simulink model "lyskawaLab6_si_nonlinear"  (R2023b)
settings: Solver=VariableStepAuto  StartTime=0.0  StopTime=stopTime  MaxStep=0.01  RelTol=1e-3
values from neighbouring files (symbols this model uses):
  A1 = 2    [lyskawaLab6.m]
  A2 = 6    [lyskawaLab6.m]
  Aw1 = 0.1 * 2    (= 0.2)    [lyskawaLab6.m]
  Aw2 = 0.1 * 6    (= 0.6)    [lyskawaLab6.m]
  dfwe1 = 0.1*fwe1max    [lyskawaLab6.m]
  dfwe2 = 0    [lyskawaLab6.m]
  fwe1_0 = arrayfwe1_0(i)    [lyskawaLab6.m]
  fwe2_0 = 0.1 * fwe2max    [lyskawaLab6.m]
  g = 9.81    [lyskawaLab6.m]
  h1_0 = fwe1_0^2/(Aw1^2 *2*g)    [lyskawaLab6.m]
  h2_0 = (fwe1_0 + fwe2_0)^2/(Aw2^2 * 2*g)    [lyskawaLab6.m]
  t0 = 5    [lyskawaLab6.m]
settings Model: Creator=aleklyskawa  LastModifiedBy=aleklyskawa

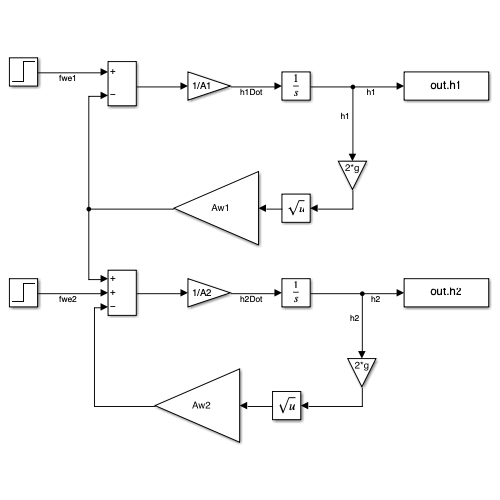
[thumbnail: Simulink's stored preview of the top-level diagram]
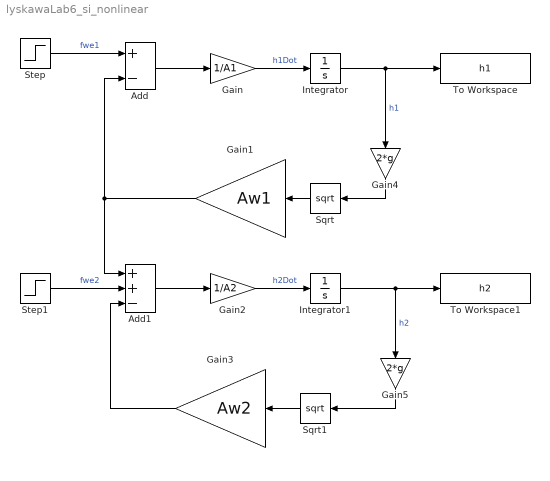
== system lyskawaLab6_si_nonlinear ==
  Add : Sum  Inputs=+-
  Add1 : Sum  Inputs=++-
  Gain : Gain  Gain=1/A1
  Gain1 : Gain  Gain=Aw1
  Gain2 : Gain  Gain=1/A2
  Gain3 : Gain  Gain=Aw2
  Gain4 : Gain  Gain=2*g
  Gain5 : Gain  Gain=2*g
  Integrator : Integrator  InitialCondition=h1_0
  Integrator1 : Integrator  InitialCondition=h2_0
  Sqrt : Sqrt
  Sqrt1 : Sqrt
  Step : Step  Time=t0  Before=fwe1_0  After=fwe1_0 + dfwe1  SampleTime=0
  Step1 : Step  Time=t0  Before=fwe2_0  After=fwe2_0 + dfwe2  SampleTime=0
  To Workspace : ToWorkspace  VariableName=h1  SampleTime=-1
  To Workspace1 : ToWorkspace  VariableName=h2  SampleTime=-1
  wires:
  Gain1/1 -> Add/2, Add1/1
  Gain2/1 -> Integrator1/1  "h2Dot"
  Add1/1 -> Gain2/1
  Integrator/1 -> Gain4/1, To Workspace/1  "h1"
  Integrator1/1 -> Gain5/1, To Workspace1/1  "h2"
  Step1/1 -> Add1/2  "fwe2"
  Gain/1 -> Integrator/1  "h1Dot"
  Add/1 -> Gain/1
  Step/1 -> Add/1  "fwe1"
  Sqrt/1 -> Gain1/1
  Sqrt1/1 -> Gain3/1
  Gain3/1 -> Add1/3
  Gain4/1 -> Sqrt/1
  Gain5/1 -> Sqrt1/1
